simulink model "sf_gfexport"  (Simulink 7.6)
settings: Solver=ode45  StartTime=0.0  StopTime=inf  RelTol=1e-3
libraries: simulink x1
settings Model: Creator=The MathWorks Inc.  CovMetricSettings=dcmtr  ExtModeAutoUpdateStatusClock=off
settings OptimizationCC: BooleanDataType=off  InlineInvariantSignals=on  InitFltsAndDblsToZero=on  EfficientMapNaN2IntZero=off
settings DebuggingCC: SaveWithParameterizedLinksMsg=none  SignalResolutionControl=TryResolveAllWithWarning  SolverPrmCheckMsg=none  MultiTaskDSMMsg=warning  MultiTaskCondExecSysMsg=none  StrictBusMsg=None
settings HardwareCC: TargetUnknown=on
settings SFSimCC: SimParseCustomCode=off
settings RTWCC: IncludeERTFirstTime=on
settings GRTTargetCC: TargetFcnLib=ansi_tfl_tmw.mat

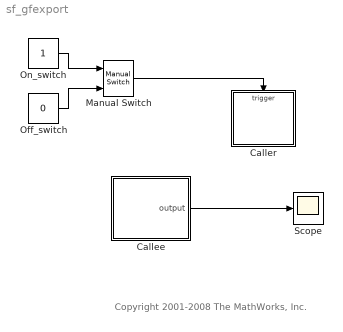
== system sf_gfexport ==
  note: Copyright 2001-2008 The MathWorks, Inc.
  Callee : Stateflow chart  TreatAsAtomicUnit=on
  Caller : Stateflow chart  TreatAsAtomicUnit=on
  Manual Switch : simulink/Signal Routing/Manual Switch  SystemSampleTime=-1  sw=0  action=0  varsize=off
  Off_switch : Constant  Value=0
  On_switch : Constant
  Scope : Scope
      settings: TimeRange=10  YMin=-1  YMax=1.3
  wires:
  On_switch/1 -> Manual Switch/1
  Off_switch/1 -> Manual Switch/2
  Manual Switch/1 -> Caller/Trigger
  Callee/1(output) -> Scope/1

== stateflow chart Caller ==
  (junction 4) -> (junction 3) [order 1] : [is_A_active()]
      | {send_event_to_A();}
  (junction 4) -> (junction 3) [order 2] : {send_event_to_B();}
  (default) -> (junction 4)
  events: E input EITHER_EDGE_EVENT

== stateflow chart Callee ==
  state A
    entry: output = 0;
  state B
    entry: output = 1;
  state activity = is_A_active() [function]
    (default) -> (junction 16) : {activity = in(A);}
  state send_event_to_A() [function]
    (default) -> (junction 17) : {send(SWITCH,A);}
  state send_event_to_B() [function]
    (default) -> (junction 18) : {send(SWITCH,B);}
  (default) -> A
  B -> A : SWITCH
  A -> B : SWITCH
  data: activity function_output double; output output double
  events: SWITCH local EITHER_EDGE_EVENT
